simulink model "EV_MAT_1"  (R2022b)
settings: Solver=FixedStepAuto  StartTime=0.0  StopTime=350  FixedStep=Ts  MaxStep=1e-3  RelTol=1e-3  EnableMultiTasking=on
PreLoadFcn:
  | ee_asm_dtc_data;
StopFcn:
  | ee_addSimlogTimeStamp(bdroot)
values from neighbouring files (symbols this model uses):
  Cap_batt = 3000    [Parametri_MODELLO_EV.m]
  fn = 60    [Parametri_MODELLO_EV.m]
  Ki_wr = 3134.24    [Parametri_MODELLO_EV.m]
  Kp_wr = 65.47    [Parametri_MODELLO_EV.m]
  p = 2    [Parametri_MODELLO_EV.m]
  pend = 0    [Parametri_MODELLO_EV.m]
  Pn = 170e3    (= 170000)    [Parametri_MODELLO_EV.m]
  psin = (Vn/sqrt(3)*sqrt(2)/wbase)    [Parametri_MODELLO_EV.m]
  Tbase = Pn/(wbase/p)    (= 901.878010854)    [Parametri_MODELLO_EV.m]
  Ts = 5e-5    (= 5e-05)    [Parametri_MODELLO_EV.m]
  Tsc = 1/(fsw*10)    (= 5e-05)    [Parametri_MODELLO_EV.m]
  Xls = Lls*Zbase    [Parametri_MODELLO_EV.m]
  z = 3    [Parametri_MODELLO_EV.m]
undefined symbols (not defined in the file or in its folder): DiscIntNeverNeededParam, ee, sigbuilder_block
libraries: nesl_utility x16, ee_lib x11, fl_lib x8, sdl_lib x7, autolibshared x2, batteryecm_lib x1, eeAsmDirectTorqueControl x1, slpidlib x1
CloseFcn:
  | clear simlog_ee_asm_dtc
  | clear logsout_ee_asm_dtc
Description:
  | Asynchronous Machine Direct Torque Control
settings Model: Creator=The MathWorks, Inc.  LastModifiedBy=Francesco Stasi
settings SolverCC: AlgebraicLoopSolver=TrustRegion  MaxZcPerStep=1
settings DataIOCC: MaxDataPoints=510000  SaveOperatingPoint=on  SaveFormat=StructureWithTime  SaveOutput=off  ReturnWorkspaceOutputs=off  SignalLoggingName=logsout_ee_asm_dtc
settings OptimizationCC: ExpressionDepthLimit=2147483647  LifeSpan=inf
settings DebuggingCC: AlgebraicLoopMsg=error  SolverPrmCheckMsg=warning  MultiTaskRateTransMsg=warning  UnconnectedInputMsg=warning  UnconnectedOutputMsg=warning  UnconnectedLineMsg=warning  StateNameClashWarn=warning  SFUnexpectedBacktrackingDiag=warning  SFNoUnconditionalDefaultTransitionDiag=warning  SFExecutionAtInitializationDiag=none  SFMachineParentedDataDiag=warning  ArithmeticOperatorsInVariantConditions=warning
settings HardwareCC: ProdBitPerPointer=32  ProdBitPerSizeT=32  ProdBitPerPtrDiffT=32  ProdLargestAtomicFloat=None  ProdIntDivRoundTo=Undefined  ProdEndianess=Unspecified  ProdWordSize=32  ProdHWDeviceType=32-bit Generic
settings ModelReferenceCC: EnableRefExpFcnMdlSchedulingChecks=on  PropagateSignalLabelsOutOfModel=off
settings SFSimCC: SimUseLocalCustomCode=off  CustomCodeUndefinedFunction=UseInterfaceOnly
settings RTWCC: RTWUseLocalCustomCode=off  DLArmComputeVersion=19.05
settings CodeAppCC: StateflowObjectComments=on
settings GRTTargetCC: TargetLangStandard=C89/C90 (ANSI)
settings ConfigComp: CovMetricSettings=dw  CovSaveCumulativeToWorkspaceVar=on  CovSaveSingleToWorkspaceVar=on  CovExternalEMLEnable=off  CovSFcnEnable=off
settings SimscapeCC: SimscapeLogType=all  SimscapeLogSimulationStatistics=on  SimscapeLogName=simlog_ee_asm_dtc  SimscapeLogDecimation=5  SimscapeLogDataHistory=510000

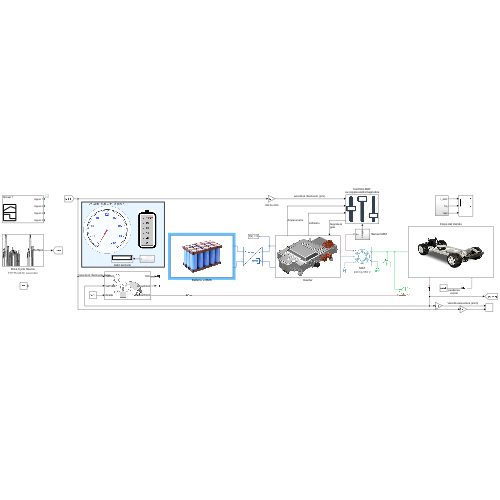
[thumbnail: Simulink's stored preview of the top-level diagram]
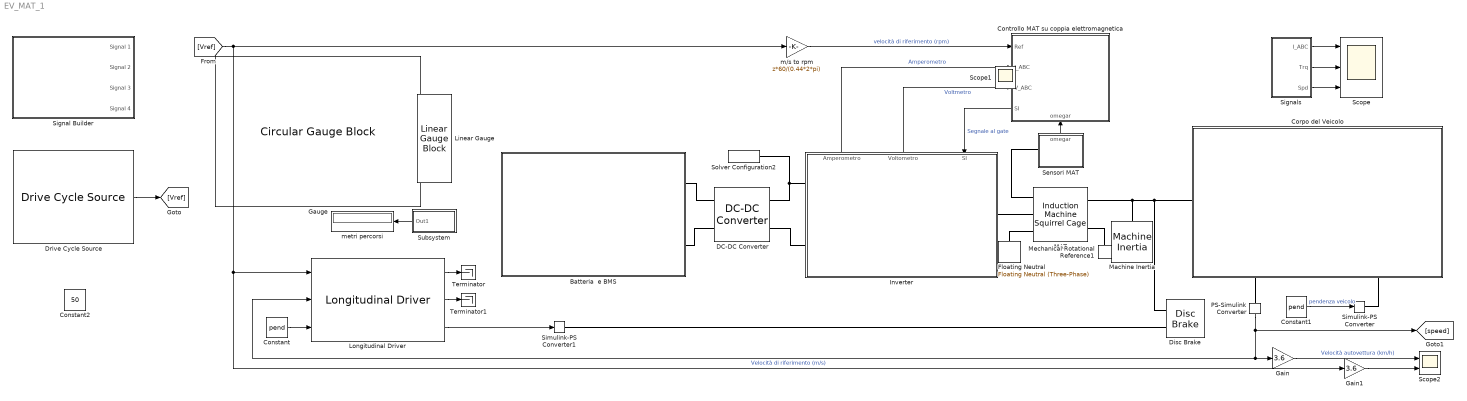
== system EV_MAT_1 ==
  Batteria  e BMS : Subsystem
      mask Display: image('C:\Users\Francesco Stasi\OneDrive\Desktop\5s3p-ifr26650-15v-9ah-lifepo4-battery-pack-cp.png'); % Use "Edit Image" on toolstrip to change.
  Constant : Constant  Value=pend
  Constant1 : Constant  Value=pend
  Constant2 : Constant  Value=50
  Controllo MAT su coppia elettromagnetica : Subsystem
      settings: PortSchema="{\"entries\":[{\"content\":{\"sides\":[{\"content\":{\"connectorIds\":[\"In1\",\"In2\",\"In3\",\"Out1\"]},\"type\":\"ConnectorPlacement.EquallySpacedRectSide\",\"uuid\":\"8f9bcb94-bb71-4a07-9882-951846ecb14c\"},{\"content\":{\"connectorIds\":[],\"side\":\"RIGHT\"},\"type\":\"ConnectorPlacement.EquallySpacedRectSide\",\"uuid\":\"e2aa7a74-1c19-4511-93dd-8eef952fef55\"},{\"content\":{\"connectorIds\":[],\"side\":\"TOP\"},\"type\":\"ConnectorPlacement.EquallySpacedRectSide\",\"uuid\":\"f6c31379-a4a6-419d-aabe-831c72e240e3\"},{\"content\":{\"connectorIds\":[\"In4\"],\"side\":\"BOTTOM\"},\"type\":\"ConnectorPlacement.EquallySpacedRectSide\",\"uuid\":\"cd6ef859-7980-4552-aa2c-c30a713633d9\"}]},\"type\":\"ConnectorPlacement.EquallySpacedConnector\",\"uuid\":\"2df81b2a-a33e-4fa2-94dc-365b63169d84\"}],\"packageUris\":[\"http://schema.mathworks.com/mf0/Connector/R2020b\"],\"version\":\"1.0\"}"
      mask Display: image('C:\Users\Francesco Stasi\Downloads\control-icon-13.jpg'); % Use "Edit Image" on toolstrip to change.
  Corpo del Veicolo : Subsystem
      settings: PortSchema="{\"entries\":[{\"content\":{\"sides\":[{\"content\":{\"connectorIds\":[\"LConn1\"]},\"type\":\"ConnectorPlacement.EquallySpacedRectSide\",\"uuid\":\"4a2885ce-fc1a-49ad-9aa6-0d3bb59923d5\"},{\"content\":{\"connectorIds\":[],\"side\":\"RIGHT\"},\"type\":\"ConnectorPlacement.EquallySpacedRectSide\",\"uuid\":\"2b1bc1ea-a3ce-42b8-a587-d0fb7b44a7f1\"},{\"content\":{\"connectorIds\":[],\"side\":\"TOP\"},\"type\":\"ConnectorPlacement.EquallySpacedRectSide\",\"uuid\":\"1b8bb2cd-3c5d-4fd3-8828-598421c59bb4\"},{\"content\":{\"connectorIds\":[\"RConn1\",\"RConn2\"],\"side\":\"BOTTOM\"},\"type\":\"ConnectorPlacement.EquallySpacedRectSide\",\"uuid\":\"393011ce-59fa-4176-b2b7-b157e857ca56\"}]},\"type\":\"ConnectorPlacement.EquallySpacedConnector\",\"uuid\":\"f348d670-56e7-4fcf-bf34-f2e47d78218d\"}],\"packageUris\":[\"http://schema.mathworks.com/mf0/Connector/R2020b\"],\"version\":\"1.0\"}"
      mask Display: image('C:\Users\Francesco Stasi\Downloads\kisspng-club-car-golf-buggies-vehicle-frame-chassis-golf-drive-5b16551246bc60.0198354915281902262897.png'); % Use "Edit Image" on toolstrip to change.
  DC-DC Converter : ee_lib/Semiconductors & Converters/Converters/DC-DC Converter  Vref_option=ee.enum.converters.voltageref.internal  v_ref=Vinv V  P_rated=1.1*Pn W  droop_enabled=true  droop_param=ee.enum.converters.droop.value  droop=0.1 V/A  droop_percent=2  Vref_droop=10 V  reversible=ee.enum.converters.directionality.unidirectional  G_diode=1e-8 1/Ohm  P_fixed=1 W  losses_option=ee.enum.converters.lossesOption.proportionalToSquaredCurrent  eff_rated=99  tableOption=ee.enum.converters.lossTableOptionThermal.currentTemp  i_eff_vec=[-2, -1, 1, 2] A  v_eff_vec=[15, 30, 45] V  eff_vec=[66, 76, 80, 74]  eff_2D_table=[66, 66, 66; 76, 76, 76; 80, 80, 80; 74, 74, 74]  model_dynamics=ee.enum.converters.dynamics.no  tau=0.02 s  v_ini=10 V  v1_min=1 V  R1=1000 Ohm  R2=1000 Ohm  enable_fault=simscape.enum.onoff.off  fault_condition=ee.enum.faults.faultInputCondition.greaterThan  fault_threshold=0.5  T_eff_vec=[280, 300, 320] K  eff_3D_table=repmat([66; 76; 80; 74], 1, 3, 3)  thermal_mass=100 J/K  initial_temperature=298.15 K
      settings: InternalSimscapePortConfiguration="{\"Bottom\":[],\"Left\":[{\"id\":\"p1\",\"label\":\"1+\",\"type\":\"foundation.electrical.electrical\"},{\"id\":\"n1\",\"label\":\"1-\",\"type\":\"foundation.electrical.electrical\"}],\"Right\":[{\"id\":\"p2\",\"label\":\"2+\",\"type\":\"foundation.electrical.electrical\"},{\"id\":\"n2\",\"label\":\"2-\",\"type\":\"foundation.electrical.electrical\"}],\"Top\":[]}"
  Disc Brake : sdl_lib/Brakes & Detents/Rotational/Disc Brake  r_mean=150 mm  bore=10 mm  n_pads=2  thermal_port=simscape.enum.thermaleffects.omit  mu_static=0.9  mu_coulomb=0.7  temperature_TLU=[280, 300, 320] K  mu_static_TLU=[.9, .8, .7]  mu_coulomb_TLU=[.8, .7, .6]  brkwy_vel=0.1 rad/s  visc_coef=0 N*m*s/rad  enable_faults=simscape.enum.onoff.off  faulted_pressure=0 bar  external_fault=simscape.enum.onoff.off  temporal_fault=simscape.enum.onoff.off  fault_time=5 s  report_fault=simscape.enum.assert.action.none  thermal_mass=50 kJ/K  temperature_specify=off  temperature_priority=High  temperature=300 K  temperature_nominal_specify=off  temperature_nominal_unit=K  temperature_nominal_value=1
  Drive Cycle Source : autolibshared/Drive Cycle Source  cycleVar=FTP75  fileVar=cycleFTP75.mat  tfinal="2474  seconds"  cycleRepeat=off  outAccPort=off  outGearPort=off  gearList=No gear data  t_wot1=5  xdot_woto=0  xdot_wot1=30  t_wot2=20  xdot_wot2=0  t_wotend=30  srcUnit=m/s  outUnit=m/s  srcAccUnit=m/s/s  outAccUnit=m/s^2  dt=0  aMode=1  faultOption=off  velBnd=2  velBndUnit=mph  inUnit=m/s  timeBnd=1  failOption=off  stopSim=off  maxFaultCnt=10  maxFaultTime=2  maxTotFaultTime=15  traceOption=off  dtTrace=1  traceWindow=10  lastDCname=FTP75  lastOutUnit=mph  lastDT=0  lastTB=1  lastSB=2  forceCalcBound=off
  Floating Neutral : ee_lib/Connectors & References/Floating Neutral (Three-Phase)  G_parasitic=1e-12 1/Ohm
      settings: InternalSimscapePortConfiguration="{\"Bottom\":[],\"Left\":[{\"id\":\"N\",\"label\":\"~\",\"type\":\"foundation.electrical.three_phase\"}],\"Right\":[],\"Top\":[]}"
  Gain : Gain  Gain=3.6
  Gain1 : Gain  Gain=3.6
  Gauge : CircularGaugeBlock  ScaleMax=240  TickInterval=30
  Inverter : Subsystem
      settings: PortSchema="{\"entries\":[{\"content\":{\"sides\":[{\"content\":{\"connectorIds\":[\"LConn1\",\"LConn2\"]},\"type\":\"ConnectorPlacement.EquallySpacedRectSide\",\"uuid\":\"85eecfe3-6ff7-4918-8110-918438e19cb0\"},{\"content\":{\"connectorIds\":[\"RConn1\"],\"side\":\"RIGHT\"},\"type\":\"ConnectorPlacement.EquallySpacedRectSide\",\"uuid\":\"4d0880c8-cc00-4cbe-898a-2bbb8d0925a5\"},{\"content\":{\"connectorIds\":[\"Out1\",\"Out2\",\"In1\"],\"side\":\"TOP\"},\"type\":\"ConnectorPlacement.EquallySpacedRectSide\",\"uuid\":\"d8ff5260-2c61-4123-82ec-e97ef69bcd79\"}]},\"type\":\"ConnectorPlacement.EquallySpacedConnector\",\"uuid\":\"f2a04f5d-6b9c-4a65-8385-a25126c73c82\"}],\"packageUris\":[\"http://schema.mathworks.com/mf0/Connector/R2020b\"],\"version\":\"1.0\"}"
      mask Display: image('C:\Users\Francesco Stasi\Downloads\inverter.png'); % Use "Edit Image" on toolstrip to change.
  Linear Gauge : LinearGaugeBlock  LabelPosition=Hide
  Longitudinal Driver : autolibshared/Longitudinal Driver  extAccelOvr=off  extDecelOvr=off  extAccelHld=off  extDecelHld=off  extAccelZero=off  extDecelZero=off  cntrlType=PI  shftType=None  velUnits=m/s  gearOut=off  Kp=15  Ki=1  Kff=.05  Kg=.01  VehVelVec=[0 100]  KffVec=[.1 .1]  KpVec=[10 10]  KiVec=[5 5]  KgVec=[0 0]  m=1500  Kpt=3000  tau=.1  L=2  aR=200  bR=2.5  cR=.5  g=9.81  vnom=100  Kaw=.1  tauerr=.03  tauPt=2  GearInit=0  tShift=.1  pdlVec=[0.1 0.4 0.5 0.9]  upShftTbl=[-1 12.9375 26.4375 39.9375 51.18749999999999 62.4375 72.84375 83.25;-1 16.3125 29.8125 43.3125 54.5624 65.8125 76.78125 87.75;-1 19.6875 33.1875 46.68749999999999 57.9375 69.1875 80.71875 92.25;-1 33 52.5 77.25 100.5 138.75 161.875 185]  dwnShftTbl=[1 9.5625 23.0625 36.5625 47.8125 59.0625 68.90625 78.75;1 12.9375 26.4375 39.9375 51.18749999999999 62.4375 72.84375 83.25;1 16.3125 29.8125 43.3125 54.562499 65.8125 76.78125 87.75;1 19.6875 33.1875 46.68749999999999 57.9375 69.1875 80.71875 92.25]  tClutch=.5  tRev=.5  tPark=120  aMode=1  UpGearVec="[0  1  2  3  4  5  6  7]"  DownGearVec="[1  2  3  4  5  6  7  8]"
  MAT : ee_lib/Electromechanical/Asynchronous/Induction Machine Squirrel Cage  port_option=ee.enum.threePhasePort.composite  SRated=Pn V*A  VRated=Vn V  FRated=fn Hz  nPolePairs=p  param_unit=ee.enum.unit.si  squirrel_cage=ee.enum.squirrelcage.Single  zero_sequence=ee.enum.park.zerosequence.include  initialization_option=ee.enum.asm.initialization.fluxvariables  Rs=Rss Ohm  Xls=Xls Ohm  pu_Rs=0.0258  pu_Lls=0.0413  Rrd=Rrr Ohm  Xlrd=Xlr Ohm  pu_Rrd=0.0145  pu_Llrd=0.0424  Rrd1=0.28 Ohm  Xlrd1=0.82 Ohm  Rrd2=0.28 Ohm  Xlrd2=0.82 Ohm  pu_Rrd1=0.0290  pu_Llrd1=0.0848  pu_Rrd2=0.0290  pu_Llrd2=0.0848  Xm=Xm Ohm  pu_Lm=1.7562  X0=Xls Ohm  pu_L0=0.0413  saturation_option=0  saturation_i=[0, 4, 9, 18, 25, 34, 50, 68, 95, 120] A  saturation_v=[0, 88, 154, 198, 220, 242, 264, 286, 308, 330] V  pu_saturation_i=[0, .176, .396, .792, 1.1, 1.496, 2.2, 2.992, 4.18, 5.28]  pu_saturation_v=[0, .4, .7, .9, 1, 1.1, 1.2, 1.3, 1.4, 1.4864]  connection_option=int32(ee.enum.Connection.delta)  angular_position_specify=off  angular_position_priority=None  angular_position=0 deg  angular_position_nominal_specify=off  angular_position_nominal_unit=deg  angular_position_nominal_value=1  pu_psids_specify=off  pu_psids_priority=None  pu_psids=0  pu_psids_nominal_specify=off  pu_psids_nominal_unit=1  pu_psids_nominal_value=1  pu_psiqs_specify=off  pu_psiqs_priority=None  pu_psiqs=0  pu_psiqs_nominal_specify=off  pu_psiqs_nominal_unit=1  pu_psiqs_nominal_value=1  pu_psi0s_specify=off  pu_psi0s_priority=None  pu_psi0s=0  pu_psi0s_nominal_specify=off  pu_psi0s_nominal_unit=1  pu_psi0s_nominal_value=1  pu_psidr_specify=off  pu_psidr_priority=None  pu_psidr=0  pu_psidr_nominal_specify=off  pu_psidr_nominal_unit=1  pu_psidr_nominal_value=1  pu_psiqr_specify=off  pu_psiqr_priority=None  pu_psiqr=0  pu_psiqr_nominal_specify=off  pu_psiqr_nominal_unit=1  pu_psiqr_nominal_value=1  pu_psidr1_specify=off  pu_psidr1_priority=None  pu_psidr1=0  pu_psidr1_nominal_specify=off  pu_psidr1_nominal_unit=1  pu_psidr1_nominal_value=1  pu_psiqr1_specify=off  pu_psiqr1_priority=None  pu_psiqr1=0  pu_psiqr1_nominal_specify=off  pu_psiqr1_nominal_unit=1  pu_psiqr1_nominal_value=1  pu_psidr2_specify=off  pu_psidr2_priority=None  pu_psidr2=0  pu_psidr2_nominal_specify=off  pu_psidr2_nominal_unit=1  pu_psidr2_nominal_value=1  pu_psiqr2_specify=off  pu_psiqr2_priority=None  pu_psiqr2=0  pu_psiqr2_nominal_specify=off  pu_psiqr2_nominal_unit=1  pu_psiqr2_nominal_value=1  psids_specify=off  psids_priority=None  psids=0 Wb  psids_nominal_specify=off  psids_nominal_unit=Wb  psids_nominal_value=1  psiqs_specify=off  psiqs_priority=None  psiqs=0 Wb  psiqs_nominal_specify=off  psiqs_nominal_unit=Wb  psiqs_nominal_value=1  psi0s_specify=off  psi0s_priority=None  psi0s=0 Wb  psi0s_nominal_specify=off  psi0s_nominal_unit=Wb  psi0s_nominal_value=1  psidr_specify=off  psidr_priority=None  psidr=0 Wb  psidr_nominal_specify=off  psidr_nominal_unit=Wb  psidr_nominal_value=1  psiqr_specify=off  psiqr_priority=None  psiqr=0 Wb  psiqr_nominal_specify=off  psiqr_nominal_unit=Wb  psiqr_nominal_value=1  psidr1_specify=off  psidr1_priority=None  psidr1=0 Wb  psidr1_nominal_specify=off  psidr1_nominal_unit=Wb  psidr1_nominal_value=1  psiqr1_specify=off  psiqr1_priority=None  psiqr1=0 Wb  psiqr1_nominal_specify=off  psiqr1_nominal_unit=Wb  psiqr1_nominal_value=1  psidr2_specify=off  psidr2_priority=None  psidr2=0 Wb  psidr2_nominal_specify=off  psidr2_nominal_unit=Wb  psidr2_nominal_value=1  psiqr2_specify=off  psiqr2_priority=None  psiqr2=0 Wb  psiqr2_nominal_specify=off  psiqr2_nominal_unit=Wb  psiqr2_nominal_value=1  slip_specify=off  slip_priority=None  slip=0  slip_nominal_specify=off  slip_nominal_unit=1  slip_nominal_value=1  real_power_generated_specify=off  real_power_generated_priority=None  real_power_generated=0 W  real_power_generated_nominal_specify=off  real_power_generated_nominal_unit=W  real_power_generated_nominal_value=1  mechanical_power_consumed_specify=off  mechanical_power_consumed_priority=None  mechanical_power_consumed=0 W  mechanical_power_consumed_nominal_specify=off  mechanical_power_consumed_nominal_unit=W  mechanical_power_consumed_nominal_value=1  Tmeas=298.15 K  alpha=3.93e-3 1/K  alpha_cage=4.4e-3 1/K  stator_thermal_mass=100 J/K  rotor_thermal_mass=200 J/K  temperatureA_specify=off  temperatureA_priority=High  temperatureA=25 degC  temperatureA_nominal_specify=off  temperatureA_nominal_unit=degC  temperatureA_nominal_value=1  temperatureB_specify=off  temperatureB_priority=High  temperatureB=25 degC  temperatureB_nominal_specify=off  temperatureB_nominal_unit=degC  temperatureB_nominal_value=1  temperatureC_specify=off  temperatureC_priority=High  temperatureC=25 degC  temperatureC_nominal_specify=off  temperatureC_nominal_unit=degC  temperatureC_nominal_value=1  temperatureR_specify=off  temperatureR_priority=High  temperatureR=25 degC  temperatureR_nominal_specify=off  temperatureR_nominal_unit=degC  temperatureR_nominal_value=1
      settings: AttributesFormatString=220 hp 550 V  InternalSimscapePortConfiguration="{\"Bottom\":[],\"Left\":[{\"id\":\"R\",\"label\":\"R\",\"type\":\"foundation.mechanical.rotational.rotational\"},{\"id\":\"C\",\"label\":\"C\",\"type\":\"foundation.mechanical.rotational.rotational\"}],\"Right\":[{\"id\":\"pu_output\",\"label\":\"pu\",\"type\":\"output\"},{\"id\":\"N1\",\"label\":\"~1\",\"type\":\"foundation.electrical.three_phase\"},{\"id\":\"N2\",\"label\":\"~2\",\"type\":\"foundation.electrical.three_phase\"}],\"Top\":[]}"
  Machine Inertia : ee_lib/Electromechanical/Mechanical/Machine Inertia  SRated=Pn V*A  FRated=fn Hz  nPolePairs=p  inertia_option=2  J=27548 kg*m^2  H=H s*W/V/A  damper_option=2  D=39.0509 N*m/(rad/s)  pu_D=F  initialization_option=2  fMechanical0=60 Hz  fElectrical0=0 Hz
      settings: InternalSimscapePortConfiguration="{\"Bottom\":[],\"Left\":[{\"id\":\"R\",\"label\":\"R\",\"type\":\"foundation.mechanical.rotational.rotational\"}],\"Right\":[],\"Top\":[]}"
  Mechanical Rotational Reference1 : fl_lib/Mechanical/Rotational Elements/Mechanical Rotational Reference
  PS-Simulink Converter : nesl_utility/PS-Simulink Converter  PhysicalDomain=network_engine_domain  SubClassName=ps_output  LeftPortType=input  RightPortType=output  PseudoPeriodic=off  Frequencies=[]  VectorFormat=inherit  Unit=inherit  AffineConversion=off
  Scope : Scope  NumInputPorts=3
  Scope2 : Scope  NumInputPorts=2
  Sensori MAT : Subsystem
      settings: PortSchema="{\"entries\":[{\"content\":{\"sides\":[{\"content\":{\"connectorIds\":[]},\"type\":\"ConnectorPlacement.EquallySpacedRectSide\",\"uuid\":\"0fbb1c44-8a9c-4a3a-ab91-37d5ce7b514b\"},{\"content\":{\"connectorIds\":[\"RConn1\"],\"side\":\"RIGHT\"},\"type\":\"ConnectorPlacement.EquallySpacedRectSide\",\"uuid\":\"48a3c917-355b-4f14-ad1c-718971ab44c8\"},{\"content\":{\"connectorIds\":[\"Out1\"],\"side\":\"TOP\"},\"type\":\"ConnectorPlacement.EquallySpacedRectSide\",\"uuid\":\"9afe0284-914f-475e-bc85-f9d1981aa904\"}]},\"type\":\"ConnectorPlacement.EquallySpacedConnector\",\"uuid\":\"87a2b5b7-2b0f-4fe2-9890-605b96c30ff6\"}],\"packageUris\":[\"http://schema.mathworks.com/mf0/Connector/R2020b\"],\"version\":\"1.0\"}"
  Signal Builder : Subsystem  Tag=STV Subsys  LoadFcn=sigbuilder_block('load');  StartFcn=sigbuilder_block('start');  StopFcn=sigbuilder_block('stop');  ClipboardFcn=sigbuilder_block('clipboard');  mask(Sigbuilder block){tuvar=[0:10]}
      mask help: Simulink:masks:SigbuilderBlock_MD
      mask init:
      | if ~strcmp(get_param(bdroot(gcbh),'SimulationStatus'),'stopped') tuvar = sigbuilder_block('maskInit'); end
      settings: CopyFcn=sigbuilder_block('copy');  DeleteFcn=sigbuilder_block('delete');  ModelCloseFcn=sigbuilder_block('modelClose');  PreSaveFcn=sigbuilder_block('preSave');  PauseFcn=sigbuilder_block('pause');  ContinueFcn=sigbuilder_block('continue');  NameChangeFcn=sigbuilder_block('namechange');  OpenFcn=sigbuilder_block('open',[150 63 720 400.5 ]);  CloseFcn=sigbuilder_block('close');
      mask Display: plot(0, 0, 100, 100,[2, 2, 32, 32, 2], [68, 8, 8, 68, 68],[32, 2], [38, 38], [32, 19, 2],[53, 60, 44], [32, 17, 17, 2],[16, 16, 31, 31]);txt = getActiveGroup(gcbh);text(2, 100, txt,'verticalAlignment', 'top');
  Signals : Subsystem
  Simulink-PS Converter : nesl_utility/Simulink-PS Converter  PhysicalDomain=network_engine_domain  SubClassName=ps_input  LeftPortType=input  RightPortType=output  PseudoPeriodic=off  Frequencies=[]  NoiseDistribution=none  NoiseParameters=[]  Unit=1  AffineConversion=off  FilteringAndDerivatives=provide  SimscapeFilterOrder=1  InputFilterTimeConstant=0.001  UdotUserProvided=0
  Simulink-PS Converter1 : nesl_utility/Simulink-PS Converter  PhysicalDomain=network_engine_domain  SubClassName=ps_input  LeftPortType=input  RightPortType=output  PseudoPeriodic=off  Frequencies=[]  NoiseDistribution=none  NoiseParameters=[]  Unit=1  AffineConversion=off  FilteringAndDerivatives=provide  SimscapeFilterOrder=1  InputFilterTimeConstant=0.001  UdotUserProvided=0
  Solver Configuration2 : nesl_utility/Solver Configuration  PhysicalDomain=network_engine_domain  SubClassName=solver  LeftPortType=input  RightPortType=generic  Tones=[]  Harmonics=[]  SimulateNoise=off  Profile=off  UseLocalSampling=off  EnableSwitchedLinearOptims=on  FrequencyDomain=off  UseCCode=off  RelTol=0.001  AbsTol=1e-06  MinStep=1e-09  ToWorkspace=off  RevertToSquareIcSolve=off  NumHomotopyIterations=100  PhasorMode=off  PhasorModeNumHarmonics=1  ConsistencySolver=NEWTON_FTOL  IndexReductionMethod=DerivativeReplacement  DoDC=off  ResidualTolerance=1e-09  ConsistencyTolSource=GLOBAL  ConsistencyAbsTol=0.001  ConsistencyRelTol=0.001  ConsistencyTolFactor=0.001  UseLocalSolver=on  LocalSolverChoice=NE_BACKWARD_EULER_ADVANCER  ResolveIndetEquations=on  FunctionEvalNumThread=1  LocalSolverSampleTime=Ts  DoFixedCost=on  MaxNonlinIter=5  MaxModeIter=2  ComputeImpulses=off  ImpulseIterations=2  LinearAlgebra=auto  LinearAlgebraNumThread=0  EquationFormulation=NE_TIME_EF  DelaysMemoryBudget=1024  AutomaticFiltering=on  FilteringTimeConstant=0.001  PartitionStorageMethod=AS_NEEDED  PartitionMemoryBudget=1024  PartitionMethod=FAST
  Subsystem : Subsystem
  Terminator : Terminator
  Terminator1 : Terminator
  m/s to rpm : Gain  Gain=z*60/(0.44*2*pi)
  metri percorsi : Display
  Scope1 : Scope
  wires:
  Signals/1(I_ABC) -> Scope/1
  Signals/2(Trq) -> Scope/2
  Signals/3(Spd) -> Scope/3
  Sensori MAT/1(omegar) -> Controllo MAT su coppia elettromagnetica/4(omegar)
  Inverter/2(Voltometro) -> Controllo MAT su coppia elettromagnetica/3(V_ABC)  "Voltmetro"
  Controllo MAT su coppia elettromagnetica/1(SI) -> Inverter/1(SI)  "Segnale al gate"
  Inverter/1(Amperometro) -> Controllo MAT su coppia elettromagnetica/2(I_ABC)  "Amperometro"
  m/s to rpm/1 -> Controllo MAT su coppia elettromagnetica/1(Ref)  "velocità di riferimento (rpm)"
  Longitudinal Driver/1 -> Terminator/1
  Longitudinal Driver/2 -> Terminator1/1
  Constant/1 -> Longitudinal Driver/3
  Constant1/1 -> Simulink-PS Converter/1  "pendenza veicolo"
  [Vref] -> Gain1/1, Longitudinal Driver/1, m/s to rpm/1  "Velocità di riferimento (m/s)"
  PS-Simulink Converter/1 -> [speed], Gain/1, Longitudinal Driver/2
  Gain1/1 -> Scope2/2
  Gain/1 -> Scope2/1  "Velocità autovettura (km/h)"
  Longitudinal Driver/3 -> Simulink-PS Converter1/1
  Subsystem/1(Out1) -> metri percorsi/1
  Drive Cycle Source/1 -> [Vref]
  connections:
  Corpo del Veicolo/LConn1 -- Disc Brake/LConn2 -- Machine Inertia/LConn1 -- MAT/LConn1
  MAT/RConn1 -- Sensori MAT/RConn1
  Mechanical Rotational Reference1/LConn1 -- MAT/LConn2
  Inverter/RConn1 -- MAT/RConn2
  Simulink-PS Converter/RConn1 -- Corpo del Veicolo/RConn2
  Floating Neutral/LConn1 -- MAT/RConn3
  PS-Simulink Converter/LConn1 -- Corpo del Veicolo/RConn1
  Inverter/LConn2 -- DC-DC Converter/RConn2
  Batteria  e BMS/LConn1 -- DC-DC Converter/LConn1
  Inverter/LConn1 -- Solver Configuration2/RConn1 -- DC-DC Converter/RConn1
  Disc Brake/LConn1 -- Simulink-PS Converter1/RConn1
  Batteria  e BMS/LConn2 -- DC-DC Converter/LConn2

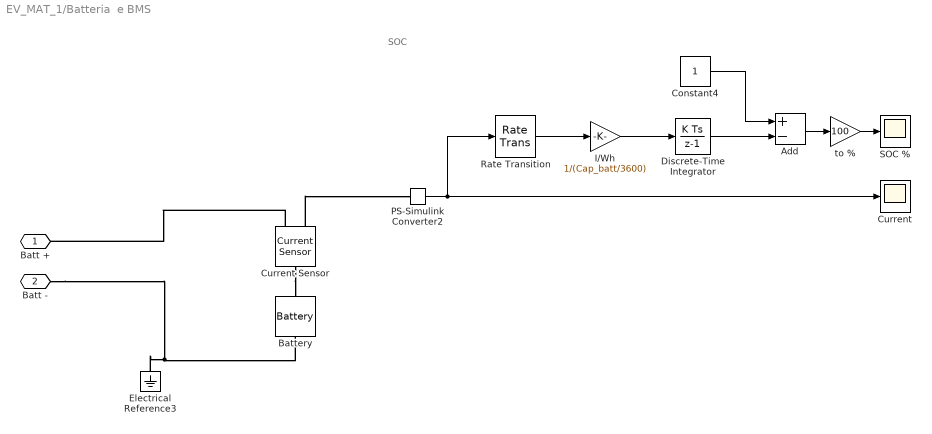
== system EV_MAT_1/Batteria  e BMS ==
  note: SOC
  Add : Sum  Inputs=+-
  Battery : batteryecm_lib/Battery  Vnom=Vbatt V  prm_dir=simscape.enum.battery.prm_dir.disabled  R1_dis=2 Ohm  R1_ch=2 Ohm  R1=2 Ohm  prm_AH=simscape.enum.battery.prm_AH.infinite  AH=50 A*hr  V1=11.5 V  AH1=25 A*hr  prm_R2=simscape.enum.battery.prm_R2.disabled  R2=2000 Ohm  prm_dyn=simscape.enum.battery.prm_dyn.off  Rp1=0.005 Ohm  tau1=30 s  Rp2=0.005 Ohm  tau2=30 s  Rp3=0.005 Ohm  tau3=30 s  Rp4=0.005 Ohm  tau4=30 s  Rp5=0.005 Ohm  tau5=30 s  prm_fade=simscape.enum.battery.prm_fade.disabled  N_fade=100  AH_fade=45 A*hr  R1_fade=2.02 Ohm  R1_ch_fade=2.02 Ohm  V1_fade=10.35 V  prm_age=simscape.enum.battery.prm_age.disabled  prm_age_OCV=simscape.enum.battery.prm_age_OCV.OCV  OCV_age=0.9  SOC_age=60  delta_time_age_vec=[0] d  temperature_age_vec=[273] K  OCV_scaling_age=2.2134e6  OCV_offset_age=1.632e6  temp_exp_age=0.515833569 V  t_exp_age=0.75  i_specify=off  i_priority=None  i=0 A  i_nominal_specify=off  i_nominal_unit=A  i_nominal_value=1  v_specify=off  v_priority=None  v=0 V  v_nominal_specify=off  v_nominal_unit=V  v_nominal_value=1  charge_specify=off  charge_priority=High  charge=50 A*hr  charge_nominal_specify=off  charge_nominal_unit=A*hr  charge_nominal_value=1  num_cycles_specify=off  num_cycles_priority=High  num_cycles=0  num_cycles_nominal_specify=off  num_cycles_nominal_unit=1  num_cycles_nominal_value=1  Tmeas=298.15 K  Tmeas_age=298.15 K  Vnom_T2=12 V  R1_T2=2.2 Ohm  R1_T2_dis=2.2 Ohm  R1_T2_ch=2.2 Ohm  V1_T2=11.4 V  R2_T2=2200 Ohm  Rp1_T2=0.005 Ohm  tau1_T2=30 s  Rp2_T2=0.005 Ohm  tau2_T2=30 s  Rp3_T2=0.005 Ohm  tau3_T2=30 s  Rp4_T2=0.005 Ohm  tau4_T2=30 s  Rp5_T2=0.005 Ohm  tau5_T2=30 s  Tmeas2=273.15 K  thermal_mass=30000 J/K  temperature_specify=off  temperature_priority=High  temperature=298.15 K  temperature_nominal_specify=off  temperature_nominal_unit=K  temperature_nominal_value=1
  Constant4 : Constant
  Current : Scope
  Current Sensor : fl_lib/Electrical/Electrical Sensors/Current Sensor
  Discrete-Time Integrator : DiscreteIntegrator  SampleTime=-1  ICPrevOutput=DiscIntNeverNeededParam  ICPrevScaledInput=DiscIntNeverNeededParam
  Electrical Reference3 : fl_lib/Electrical/Electrical Elements/Electrical Reference
  I/Wh : Gain  Gain=1/(Cap_batt/3600)
  PS-Simulink Converter2 : nesl_utility/PS-Simulink Converter  PhysicalDomain=network_engine_domain  SubClassName=ps_output  LeftPortType=input  RightPortType=output  PseudoPeriodic=off  Frequencies=[]  VectorFormat=1-D array  Unit=inherit  AffineConversion=off
  Rate Transition : RateTransition
  SOC % : Scope
  to % : Gain  Gain=100
  Batt + : PMIOPort  Side=Left
  Batt - : PMIOPort  Port=2  Side=Left
  wires:
  PS-Simulink Converter2/1 -> Rate Transition/1, Current/1
  Constant4/1 -> Add/1
  I/Wh/1 -> Discrete-Time Integrator/1
  Rate Transition/1 -> I/Wh/1
  Discrete-Time Integrator/1 -> Add/2
  Add/1 -> to %/1
  to %/1 -> SOC %/1
  connections:
  Current Sensor/RConn1 -- PS-Simulink Converter2/LConn1
  Current Sensor/RConn2 -- Batt +/RConn1
  Current Sensor/LConn1 -- Battery/LConn1
  Batt -/RConn1 -- Electrical Reference3/LConn1 -- Battery/RConn1

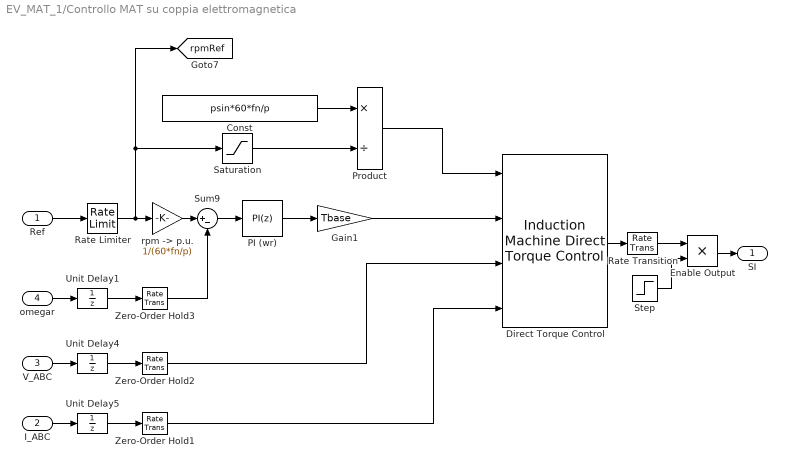
== system EV_MAT_1/Controllo MAT su coppia elettromagnetica ==
  Ref : Inport
  I_ABC : Inport  Port=2
  V_ABC : Inport  Port=3
  omegar : Inport  Port=4
  " Direct Torque Control" : eeAsmDirectTorqueControl/Induction Machine Direct Torque Control  Rs=Rss  p=p  FluxHystBand=0.2  THystBand=100  Ts=Tsc
  Const : Constant  Value=psin*60*fn/p
  Enable Output : Product
  Gain1 : Gain  Gain=Tbase
  PI (wr) : slpidlib/PID Controller  Controller=PI  Form=Parallel  TimeDomain=Discrete-time  UseExternalTs=off  SampleTime=Tsc  IntegratorMethod=Forward Euler  FilterMethod=Forward Euler  ControllerParametersSource=internal  P=Kp_wr  I=Ki_wr  UseKiTs=off  D=0  N=100  UseFilter=on  TunerSelectOption=Transfer Function Based (PID Tuner App)  InitialConditionSource=internal  InitialConditionForIntegrator=0  InitialConditionForFilter=0  DifferentiatorICPrevScaledInput=0  ExternalReset=none  TrackingMode=off  Kt=1  LimitOutput=on  SatLimitsSource=internal  UpperSaturationLimit=2  LowerSaturationLimit=-2  LinearizeAsGain=on  AntiWindupMode=back-calculation  Kb=1000  LimitIntegrator=off  UpperIntegratorSaturationLimit=inf  LowerIntegratorSaturationLimit=-inf  POutMin=[]  POutMax=[]  IOutMin=[]  IOutMax=[]  DOutMin=[]  DOutMax=[]  NOutMin=[]  NOutMax=[]  SumOutMin=[]  SumOutMax=[]  SaturationOutMin=[]  SaturationOutMax=[]  PParamMin=[]  PParamMax=[]  IParamMin=[]  IParamMax=[]  DParamMin=[]  DParamMax=[]  NParamMin=[]  NParamMax=[]  KbParamMin=[]  KbParamMax=[]  KtParamMin=[]  KtParamMax=[]  KbOutMin=[]  KbOutMax=[]  KtOutMin=[]  KtOutMax=[]  IntegratorOutMin=[]  IntegratorOutMax=[]  FilterOutMin=[]  FilterOutMax=[]  SumI1OutMin=[]  SumI1OutMax=[]  SumI2OutMin=[]  SumI2OutMax=[]  SumI3OutMin=[]  SumI3OutMax=[]  SumI4OutMin=[]  SumI4OutMax=[]  SumDOutMin=[]  SumDOutMax=[]  DifferentiatorOutMin=[]  DifferentiatorOutMax=[]  FilterDiffOutCoefMin=[]  FilterDiffOutCoefMax=[]  ReciprocalOutMin=[]  ReciprocalOutMax=[]  SumDenOutMin=[]  SumDenOutMax=[]  SumNumOutMin=[]  SumNumOutMax=[]  DivideOutMin=[]  DivideOutMax=[]  UdiffTsProdOutMin=[]  UdiffTsProdOutMax=[]  NTsProdOutMin=[]  NTsProdOutMax=[]  UintegralTsProdOutMin=[]  UintegralTsProdOutMax=[]  UngainTsProdOutMin=[]  UngainTsProdOutMax=[]  ClampingZeroOutDataTypeStr=Inherit: Inherit via back propagation  ClampingZeroOutMin=[]  ClampingZeroOutMax=[]  FilterDenConstantOutDataTypeStr=Inherit: Inherit via back propagation  FilterDenConstantOutMin=[]  FilterDenConstantOutMax=[]  PCopyOutDataTypeStr=Inherit: Inherit via back propagation  PCopyOutMin=[]  PCopyOutMax=[]  NCopyOutDataTypeStr=Inherit: Inherit via back propagation  NCopyOutMin=[]  NCopyOutMax=[]  IntegratorContinuousStateAttributes=''  IntegratorStateMustResolveToSignalObject=off  IntegratorRTWStateStorageClass=Auto  FilterContinuousStateAttributes=''  FilterStateMustResolveToSignalObject=off  FilterRTWStateStorageClass=Auto  ParallelPVariant=InternalParameters  IdealPVariant=Disabled  IVariant=InternalParameters  DVariant=Disabled  IntegratorVariant=Discrete  SatVariant=Enabled  AWVariant=BackCalculation  PCopyVariant=Disabled  TRVariant=Disabled  FdbkBlocksVariant=Forward  IdealPFdbkVariant=Disabled  SatFdbkVariant=Disabled  DerivativeFilterVariant=Disabled  NVariant=Disabled  NCopyVariant=Disabled_SignalSpec  FilterICVariant=Disabled  IntegratorICVariant=InternalICs  ExternalResetVariant=Disabled  TRSumVariant=Passthrough  SumFdbkVariant=Disabled  SumVariant=Sum_PI  TsampFilterVariant=InternalTs  TsampNgainVariant=Passthrough  TsampIntegralVariant=Passthrough  ExternalSaturationOutDataTypeStr=Inherit: Same as second input
  Product : Product  Inputs=*/
  Rate Limiter : RateLimiter  RisingSlewLimit=2000  FallingSlewLimit=-2000  SampleTimeMode=inherited
      settings: AttributesFormatString=%<RisingSlewLimit> rpm/s
  Rate Transition : RateTransition
  Saturation : Saturate  UpperLimit=inf  LowerLimit=60*fn/p
  Step : Step  Time=0.1  SampleTime=Ts
      settings: AttributesFormatString=%<After> at %<Time> s
  Sum9 : Sum  Inputs=|+-
  Unit Delay1 : UnitDelay  SampleTime=Ts  HasFrameUpgradeWarning=on
  Unit Delay4 : UnitDelay  SampleTime=Ts  HasFrameUpgradeWarning=on
  Unit Delay5 : UnitDelay  SampleTime=Ts  HasFrameUpgradeWarning=on
  Zero-Order Hold1 : RateTransition  OutPortSampleTime=5e-05
  Zero-Order Hold2 : RateTransition  OutPortSampleTime=5e-05
  Zero-Order Hold3 : RateTransition  OutPortSampleTime=5e-05
  "rpm -> p.u." : Gain  Gain=1/(60*fn/p)
  SI : Outport  VectorParamsAs1DForOutWhenUnconnected=off
  tag scope: rpmRef=global
  wires:
  Gain1/1 -> " Direct Torque Control"/2
  Step/1 -> Enable Output/2
  Sum9/1 -> PI (wr)/1
  "rpm -> p.u."/1 -> Sum9/1
  Zero-Order Hold1/1 -> " Direct Torque Control"/4
  Unit Delay1/1 -> Zero-Order Hold3/1
  Zero-Order Hold2/1 -> " Direct Torque Control"/3
  PI (wr)/1 -> Gain1/1
  Zero-Order Hold3/1 -> Sum9/2
  Enable Output/1 -> SI/1
  V_ABC/1 -> Unit Delay4/1
  Rate Transition/1 -> Enable Output/1
  omegar/1 -> Unit Delay1/1
  Unit Delay5/1 -> Zero-Order Hold1/1
  Unit Delay4/1 -> Zero-Order Hold2/1
  " Direct Torque Control"/1 -> Rate Transition/1
  I_ABC/1 -> Unit Delay5/1
  Const/1 -> Product/1
  Saturation/1 -> Product/2
  Product/1 -> " Direct Torque Control"/1
  Ref/1 -> Rate Limiter/1
  Rate Limiter/1 -> [rpmRef], Saturation/1, "rpm -> p.u."/1

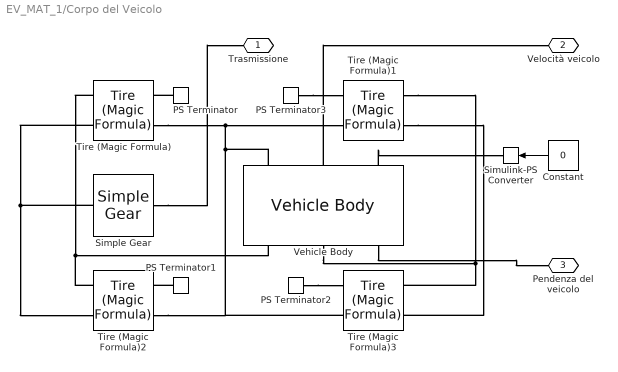
== system EV_MAT_1/Corpo del Veicolo ==
  Constant : Constant  Value=0
  PS Terminator{,1..3} (4 alike) : fl_lib/Physical Signals/Sinks/PS Terminator
  Simple Gear : sdl_lib/Gears/Simple Gear  ratio=z  rotation_direction=sdl.enum.shaftOutputDirection.same  friction_model=sdl.enum.gear_efficiencies_load.off  T_noload=0.1 N*m  T_nom=5 N*m  efficiency_nom=0.8  efficiency=0.8  temperature_TLU=[280, 300, 320] K  load_TLU=[1, 5, 10] N*m  efficiency_TLU=[.95, .9, .85]  efficiency_TLU2=[.85, .8, .75; .95, .9, .85; .85, .8, .7]  w_thr=0.01 rad/s  pwr_thr=0.001 W  backlash_model=sdl.enum.backlashModel.Off  backlash_distance=1e-3 mm  x0=0 mm  r_base=0.1 m  hardstop_model=simscape.enum.hardstop.smooth  transition=1e-4 mm  backlash_stiffness=1e7 N/m  backlash_damping=1e6 N*s/m  e=0  v_tol=0.001 m/s  mu_visc=[0, 0] N*m*s/rad  enable_faults=simscape.enum.onoff.off  efficiency_fault=0.05  external_fault=simscape.enum.onoff.off  temporal_fault=simscape.enum.onoff.off  fault_time=5 s  fault_angles=pi / 12 rad  report_fault=simscape.enum.assert.action.none  thermal_mass=50 J/K  temperature_specify=off  temperature_priority=High  temperature=300 K  temperature_nominal_specify=off  temperature_nominal_unit=K  temperature_nominal_value=1  x_backlash_specify=off  x_backlash_priority=None  x_backlash=0 mm  x_backlash_nominal_specify=off  x_backlash_nominal_unit=mm  x_backlash_nominal_value=1  f_hardstop_specify=off  f_hardstop_priority=None  f_hardstop=0 N  f_hardstop_nominal_specify=off  f_hardstop_nominal_unit=N  f_hardstop_nominal_value=1  v_backlash_specify=off  v_backlash_priority=None  v_backlash=0 m/s  v_backlash_nominal_specify=off  v_backlash_nominal_unit=m/s  v_backlash_nominal_value=1
  Simulink-PS Converter : nesl_utility/Simulink-PS Converter  PhysicalDomain=network_engine_domain  SubClassName=ps_input  LeftPortType=input  RightPortType=output  PseudoPeriodic=off  Frequencies=[]  NoiseDistribution=none  NoiseParameters=[]  Unit=1  AffineConversion=off  FilteringAndDerivatives=provide  SimscapeFilterOrder=1  InputFilterTimeConstant=0.001  UdotUserProvided=0
  Tire (Magic Formula){,1..3} (4 alike) : sdl_lib/Tires & Vehicles/Tire (Magic Formula)  parameterization=sdl.enum.magic_tire_model.peak  F_z1=3000 N  F_x1=3500 N  kappa1=10  B_m=10  C_m=1.9  D_m=1  E_m=0.97  fz0=4000 N  p_Cx=1.685  p_Dx=[1.21, -.037]  p_Ex=[.344, .095, -.02, 0]  p_Kx=[21.51, -.163, .245]  p_Hx=[-.002, .002]  p_Vx=[0, 0]  r_e=R m  model_compliance=sdl.enum.compliance.off  stiffness=1e6 N/m  damping=1000 N*s/m  model_inertia=sdl.enum.model_inertia.off  inertia=1 kg*m^2  initial_velocity=0 rad/s  model_resistance=simscape.enum.onoff.off  resistance_model=sdl.enum.rollingResistanceParameterization.constant  coeff=0.015  p_tire=250e3 Pa  alpha=-0.003  beta=0.97  coeff_a=84e-4  coeff_b=6.2e-4 s/m  coeff_c=1.6e-4 s^2/m^2  v_thr=0.001 m/s  v_tr_thr=0.1 m/s
  Vehicle Body : sdl_lib/Tires & Vehicles/Vehicle Body  mass=M kg  n_w=2  x_f=1.4 m  x_r=1.6 m  y_c=0.5 m  mass_var=simscape.enum.onoff.off  g=9.81 m/s^2  liftoff_warning=simscape.enum.onoff.off  area=3 m^2  Cd=0.4  rho=1.16 kg/m^3  model_pitch=simscape.enum.onoff.on  inertia=4000 kg*m^2  suspension_model=sdl.enum.linearTLU.linear  k_f=1e4 N/m  b_f=1e4 N*s/m  k_r=1e4 N/m  b_r=1e4 N*s/m  k_f_TLU=[-2000, -1000, 0, 1000, 2000] N  x_f_TLU=[-.4, -.2, 0, .2, .4] m  b_f_TLU=[-200, -100, 0, 100, 200] N  v_f_TLU=[-4, -2, 0, 2, 4] m/s  k_r_TLU=[-2000, -1000, 0, 1000, 2000] N  x_r_TLU=[-.4, -.2, 0, .2, .4] m  b_r_TLU=[-200, -100, 0, 100, 200] N  v_r_TLU=[-4, -2, 0, 2, 4] m/s  interp_method=simscape.enum.interpolation.linear  extrap_method=simscape.enum.extrapolation.linear  model_hardstop=simscape.enum.onoff.off  upper_bound_f=.25 m  lower_bound_f=-.25 m  stop_k_f=1e6 N/m  stop_b_f=150 N*s/m  upper_bound_r=.25 m  lower_bound_r=-.25 m  stop_k_r=1e6 N/m  stop_b_r=150 N*s/m  initial_pitch=0 rad  initial_pitch_rate=0 rad/s  v_specify=off  v_priority=High  v=0 m/s  v_nominal_specify=off  v_nominal_unit=m/s  v_nominal_value=1
  Trasmissione : PMIOPort  Side=Left
  Velocità veicolo : PMIOPort  Port=2  Side=Right
  Pendenza del veicolo : PMIOPort  Port=3  Side=Right
  wires:
  Constant/1 -> Simulink-PS Converter/1
  connections:
  Tire (Magic Formula)/RConn2 -- Vehicle Body/LConn1 -- Tire (Magic Formula)2/RConn2 -- Tire (Magic Formula)3/RConn2 -- Tire (Magic Formula)1/RConn2
  Tire (Magic Formula)/LConn2 -- Tire (Magic Formula)2/LConn2 -- Simple Gear/RConn1
  Tire (Magic Formula)2/LConn1 -- Tire (Magic Formula)/LConn1 -- Vehicle Body/RConn1
  Vehicle Body/RConn2 -- Tire (Magic Formula)1/LConn1 -- Tire (Magic Formula)3/LConn1
  Vehicle Body/RConn3 -- Pendenza del veicolo/RConn1
  Tire (Magic Formula)1/LConn2 -- Tire (Magic Formula)3/LConn2
  Vehicle Body/LConn3 -- Simulink-PS Converter/RConn1
  Vehicle Body/LConn2 -- Velocità veicolo/RConn1
  Simple Gear/LConn1 -- Trasmissione/RConn1
  PS Terminator/LConn1 -- Tire (Magic Formula)/RConn1
  PS Terminator1/LConn1 -- Tire (Magic Formula)2/RConn1
  PS Terminator2/LConn1 -- Tire (Magic Formula)3/RConn1
  PS Terminator3/LConn1 -- Tire (Magic Formula)1/RConn1

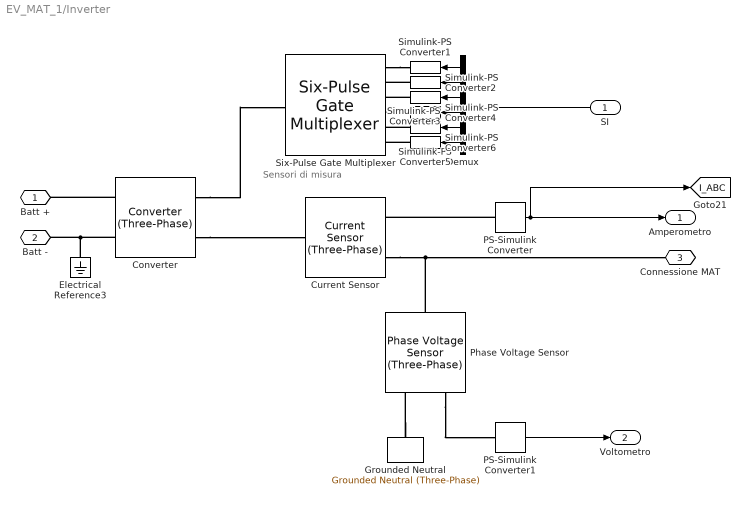
== system EV_MAT_1/Inverter ==
  note: Sensori di misura
  SI : Inport
  Converter : ee_lib/Semiconductors & Converters/Converters/Converter (Three-Phase)  port_option=ee.enum.threePhasePort.composite  device_type=3  K=0  Vf=0.8 V  Ron=0.001 Ohm  Rds=0.001 Ohm  Goff=1e-5 1/Ohm  Vgt=1 V  Vgt_off=-1 V  Ih=1 A  Vth=0.5 V  diode_param=2  diode_Vf=0.8 V  diode_Ron=0.001 Ohm  diode_Goff=1e-5 1/Ohm  diode_C=50 nF  diode_iRM=-235 A  diode_iF=300 A  diode_idot=-50 A/us  diode_trr_param=1  diode_trr_factor=3  diode_trr=15 us  diode_Qrr=1.5e+3 s*uA  snubber_type=0  Cs=1e-7 F  Rs=0.1 Ohm
  Current Sensor : ee_lib/Sensors & Transducers/Current Sensor (Three-Phase)
  Demux : Demux  Outputs=6
  Electrical Reference3 : fl_lib/Electrical/Electrical Elements/Electrical Reference
  Grounded Neutral : ee_lib/Connectors & References/Grounded Neutral (Three-Phase)
  PS-Simulink Converter : nesl_utility/PS-Simulink Converter  PhysicalDomain=network_engine_domain  SubClassName=ps_output  LeftPortType=input  RightPortType=output  PseudoPeriodic=off  Frequencies=[]  VectorFormat=1-D array  Unit=A  AffineConversion=off
  PS-Simulink Converter1 : nesl_utility/PS-Simulink Converter  PhysicalDomain=network_engine_domain  SubClassName=ps_output  LeftPortType=input  RightPortType=output  PseudoPeriodic=off  Frequencies=[]  VectorFormat=1-D array  Unit=V  AffineConversion=off
  Phase Voltage Sensor : ee_lib/Sensors & Transducers/Phase Voltage Sensor (Three-Phase)
  Simulink-PS Converter{1..6} (6 alike) : nesl_utility/Simulink-PS Converter  PhysicalDomain=network_engine_domain  SubClassName=ps_input  LeftPortType=input  RightPortType=output  PseudoPeriodic=off  Frequencies=[]  NoiseDistribution=none  NoiseParameters=[]  Unit=1  AffineConversion=off  FilteringAndDerivatives=zero  SimscapeFilterOrder=1  InputFilterTimeConstant=0.001  UdotUserProvided=1
  Six-Pulse Gate Multiplexer : ee_lib/Semiconductors & Converters/Converters/Six-Pulse Gate Multiplexer  port_option=ee.enum.controlport.ps
  Batt + : PMIOPort  Side=Left
  Batt - : PMIOPort  Port=2  Side=Left
  Connessione MAT : PMIOPort  Port=3  Side=Right
  Amperometro : Outport
  Voltometro : Outport  Port=2
  tag scope: I_ABC=global
  wires:
  PS-Simulink Converter1/1 -> Voltometro/1
  Demux/4 -> Simulink-PS Converter4/1
  Demux/1 -> Simulink-PS Converter1/1
  Demux/6 -> Simulink-PS Converter6/1
  Demux/3 -> Simulink-PS Converter3/1
  Demux/2 -> Simulink-PS Converter2/1
  Demux/5 -> Simulink-PS Converter5/1
  SI/1 -> Demux/1
  PS-Simulink Converter/1 -> [I_ABC], Amperometro/1
  connections:
  Simulink-PS Converter4/RConn1 -- Six-Pulse Gate Multiplexer/LConn4
  Phase Voltage Sensor/LConn1 -- Connessione MAT/RConn1 -- Current Sensor/RConn2
  Grounded Neutral/LConn1 -- Phase Voltage Sensor/RConn2
  Simulink-PS Converter3/RConn1 -- Six-Pulse Gate Multiplexer/LConn3
  Phase Voltage Sensor/RConn1 -- PS-Simulink Converter1/LConn1
  PS-Simulink Converter/LConn1 -- Current Sensor/RConn1
  Simulink-PS Converter5/RConn1 -- Six-Pulse Gate Multiplexer/LConn5
  Simulink-PS Converter6/RConn1 -- Six-Pulse Gate Multiplexer/LConn6
  Simulink-PS Converter2/RConn1 -- Six-Pulse Gate Multiplexer/LConn2
  Six-Pulse Gate Multiplexer/LConn1 -- Simulink-PS Converter1/RConn1
  Converter/RConn2 -- Electrical Reference3/LConn1 -- Batt -/RConn1
  Converter/RConn1 -- Batt +/RConn1
  Converter/LConn2 -- Current Sensor/LConn1
  Converter/LConn1 -- Six-Pulse Gate Multiplexer/RConn1

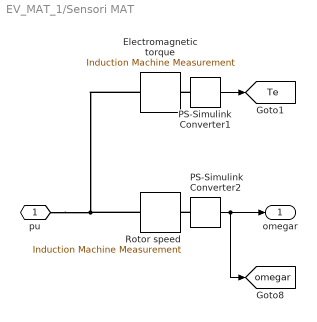
== system EV_MAT_1/Sensori MAT ==
  Electromagnetic torque : ee_lib/Electromechanical/Asynchronous/Induction Machine Measurement  output_idx=1
      settings: InternalSimscapePortConfiguration="{\"Bottom\":[],\"Left\":[{\"id\":\"pu_input\",\"label\":\"pu\",\"type\":\"input\"}],\"Right\":[{\"id\":\"pu_output\",\"label\":\"o\",\"type\":\"output\"}],\"Top\":[]}"
  PS-Simulink Converter1 : nesl_utility/PS-Simulink Converter  PhysicalDomain=network_engine_domain  SubClassName=ps_output  LeftPortType=input  RightPortType=output  PseudoPeriodic=off  Frequencies=[]  VectorFormat=1-D array  Unit=1  AffineConversion=off
  PS-Simulink Converter2 : nesl_utility/PS-Simulink Converter  PhysicalDomain=network_engine_domain  SubClassName=ps_output  LeftPortType=input  RightPortType=output  PseudoPeriodic=off  Frequencies=[]  VectorFormat=1-D array  Unit=1  AffineConversion=off
  Rotor speed : ee_lib/Electromechanical/Asynchronous/Induction Machine Measurement  output_idx=2
      settings: InternalSimscapePortConfiguration="{\"Bottom\":[],\"Left\":[{\"id\":\"pu_input\",\"label\":\"pu\",\"type\":\"input\"}],\"Right\":[{\"id\":\"pu_output\",\"label\":\"o\",\"type\":\"output\"}],\"Top\":[]}"
  pu : PMIOPort  Side=Right
  omegar : Outport
  tag scope: Te=global, omegar=global
  wires:
  PS-Simulink Converter2/1 -> omegar/1, [omegar]
  PS-Simulink Converter1/1 -> [Te]
  connections:
  PS-Simulink Converter2/LConn1 -- Rotor speed/RConn1
  PS-Simulink Converter1/LConn1 -- Electromagnetic torque/RConn1
  Electromagnetic torque/LConn1 -- pu/RConn1 -- Rotor speed/LConn1

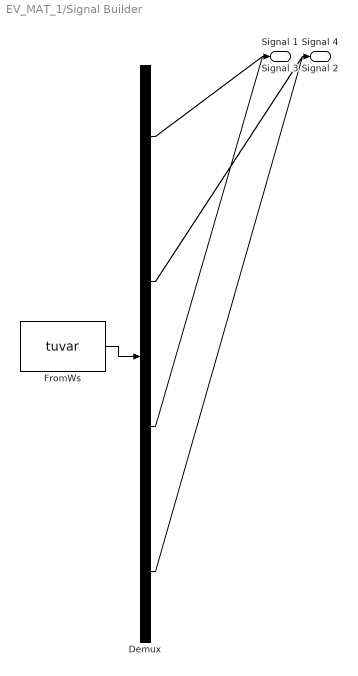
== system EV_MAT_1/Signal Builder ==
  Demux : Demux  Tag=STV Demux
      settings: DisplayOption=none
  FromWs : FromWorkspace  Tag=STV FromWs  VariableName=tuvar
      SigBuilderData=|
      | common.afterFinalStr = 'Extrapolate'
      | common.sampleTime = 0
      | dataSet.timeRange = [0 20]
      | dataSet.name = 'Group 1'
      | sbobj.Groups.Name = 'Group 1'
      | sbobj.Groups.Signals(1).Name = 'Signal 1'
      | sbobj.Groups.Signals(1).XData = [0 20]
      | sbobj.Groups.Signals(1).YData = [0.4 30.4]
      | sbobj.Groups.Signals(2).Name = 'Signal 2'
      | sbobj.Groups.Signals(2).XData = [0 20]
      | sbobj.Groups.Signals(2).YData = [0 0]
      | sbobj.Groups.Signals(3).Name = 'Signal 3'
      | sbobj.Groups.Signals(3).XData = [0 10 20]
      | sbobj.Groups.Signals(3).YData = [0 1 0.54]
      | sbobj.Groups.Signals(4).Name = 'Signal 4'
      | sbobj.Groups.Signals(4).XData = [0 8 12 12 20]
      | sbobj.Groups.Signals(4).YData = [0 30 30 0 0]
      | sbobj.Groups.TimeRange = [0 20]
  Signal 1 : Outport  Tag=STV Outport
  Signal 2 : Outport  Tag=STV Outport  Port=2
  Signal 3 : Outport  Tag=STV Outport  Port=3
  Signal 4 : Outport  Tag=STV Outport  Port=4
  wires:
  FromWs/1 -> Demux/1
  Demux/1 -> Signal 1/1
  Demux/2 -> Signal 2/1
  Demux/3 -> Signal 3/1
  Demux/4 -> Signal 4/1

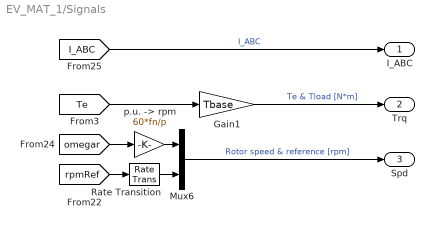
== system EV_MAT_1/Signals ==
  Gain1 : Gain  Gain=Tbase
  Mux6 : Mux  Inputs=2
  Rate Transition : RateTransition
  "p.u. -> rpm" : Gain  Gain=60*fn/p
  I_ABC : Outport  VectorParamsAs1DForOutWhenUnconnected=off
  Trq : Outport  Port=2  VectorParamsAs1DForOutWhenUnconnected=off
  Spd : Outport  Port=3  VectorParamsAs1DForOutWhenUnconnected=off
  wires:
  [omegar] -> "p.u. -> rpm"/1
  Mux6/1 -> Spd/1  "Rotor speed & reference [rpm]"
  "p.u. -> rpm"/1 -> Mux6/1
  [rpmRef] -> Rate Transition/1
  Rate Transition/1 -> Mux6/2
  [I_ABC] -> I_ABC/1  "I_ABC"
  [Te] -> Gain1/1
  Gain1/1 -> Trq/1  "Te & Tload [N*m]"

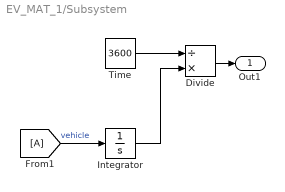
== system EV_MAT_1/Subsystem ==
  Divide : Product  Inputs=/*
  From1 : From
  Integrator : Integrator
  Time : Constant  Value=3600
  Out1 : Outport
  wires:
  Divide/1 -> Out1/1
  From1/1 -> Integrator/1  "vehicle"
  Time/1 -> Divide/1
  Integrator/1 -> Divide/2
